simulink model "gm_DUALportRAMinterface_vnl"  (R2024a)
settings: Solver=FixedStepDiscrete  StartTime=0.0  StopTime=2  RelTol=1e-3
undefined symbols (not defined in the file or in its folder): Ts
libraries: hdlsllib x18, simulink x5
settings Model: Creator=Simon  LastModifiedBy=Simon
settings OptimizationCC: BlockReduction=off  ConditionallyExecuteInputs=off  DefaultParameterBehavior=Inlined  InheritOutputTypeSmallerThanSingle=on
settings DebuggingCC: AlgebraicLoopMsg=error  InheritedTsInSrcMsg=none  SingleTaskRateTransMsg=error  UnconnectedInputMsg=warning  UnconnectedOutputMsg=warning  UnconnectedLineMsg=warning
settings HardwareCC: ProdBitPerPointer=32  ProdBitPerSizeT=32  ProdBitPerPtrDiffT=32  ProdLargestAtomicFloat=None  ProdIntDivRoundTo=Undefined  ProdEndianess=Unspecified  ProdWordSize=32  ProdHWDeviceType=ASIC/FPGA->ASIC/FPGA  TargetBitPerPointer=64  TargetBitPerSizeT=64  TargetBitPerPtrDiffT=64  TargetLongLongMode=on  TargetIntDivRoundTo=Zero  TargetEndianess=LittleEndian  TargetWordSize=64  TargetHWDeviceType=Custom Processor->MATLAB Host Computer  ProdEqTarget=off

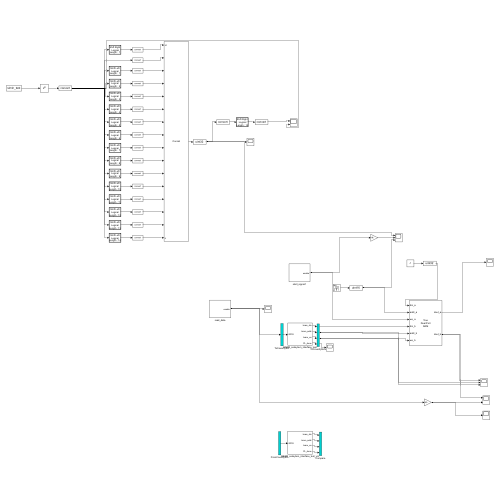
[thumbnail: Simulink's stored preview of the top-level diagram]
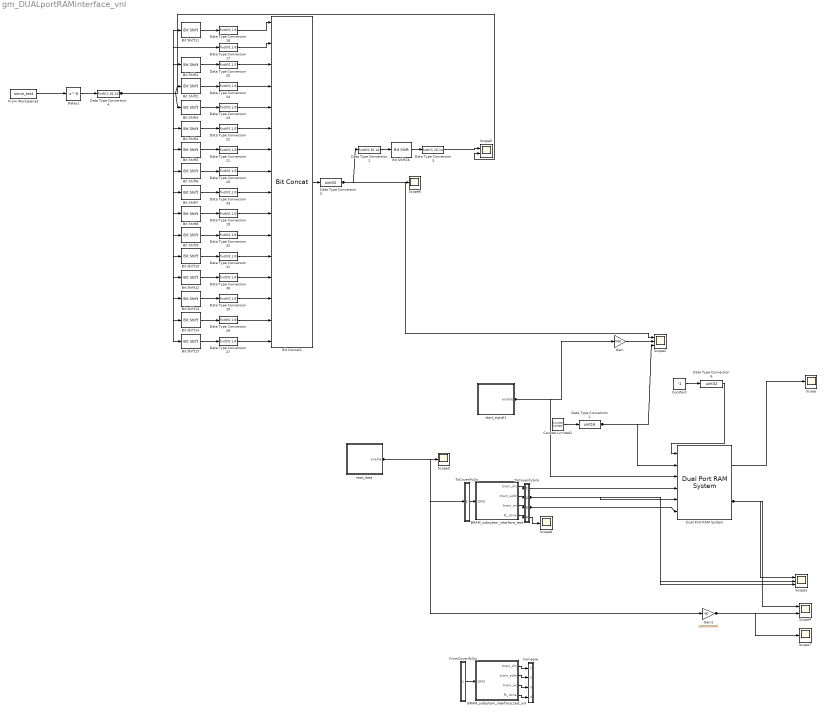
== system gm_DUALportRAMinterface_vnl ==
  BRAM_subsytem_interface_test : Subsystem
  BRAM_subsytem_interface_test_vnl : Subsystem
  Bit Concat1 : hdlsllib/Logic and Bit Operations/Bit Concat  numInputs=16
  Bit Shift1 : hdlsllib/Logic and Bit Operations/Bit Shift  mode=Shift Left Logical  N=1
  Bit Shift10 : hdlsllib/Logic and Bit Operations/Bit Shift  mode=Shift Left Logical  N=10
  Bit Shift11 : hdlsllib/Logic and Bit Operations/Bit Shift  mode=Shift Right Logical  N=1
  Bit Shift12 : hdlsllib/Logic and Bit Operations/Bit Shift  mode=Shift Left Logical  N=11
  Bit Shift13 : hdlsllib/Logic and Bit Operations/Bit Shift  mode=Shift Left Logical  N=12
  Bit Shift14 : hdlsllib/Logic and Bit Operations/Bit Shift  mode=Shift Left Logical  N=13
  Bit Shift15 : hdlsllib/Logic and Bit Operations/Bit Shift  mode=Shift Left Logical  N=14
  Bit Shift16 : hdlsllib/Logic and Bit Operations/Bit Shift  mode=Shift Right Logical  N=14
  Bit Shift2 : hdlsllib/Logic and Bit Operations/Bit Shift  mode=Shift Left Logical  N=2
  Bit Shift3 : hdlsllib/Logic and Bit Operations/Bit Shift  mode=Shift Left Logical  N=3
  Bit Shift4 : hdlsllib/Logic and Bit Operations/Bit Shift  mode=Shift Left Logical  N=4
  Bit Shift5 : hdlsllib/Logic and Bit Operations/Bit Shift  mode=Shift Left Logical  N=5
  Bit Shift6 : hdlsllib/Logic and Bit Operations/Bit Shift  mode=Shift Left Logical  N=6
  Bit Shift7 : hdlsllib/Logic and Bit Operations/Bit Shift  mode=Shift Left Logical  N=7
  Bit Shift8 : hdlsllib/Logic and Bit Operations/Bit Shift  mode=Shift Left Logical  N=8
  Bit Shift9 : hdlsllib/Logic and Bit Operations/Bit Shift  mode=Shift Left Logical  N=9
  Compare : Subsystem
      mask Display: disp('')
  Constant : Constant  Value=-1  SampleTime=-1
  Counter Limited1 : simulink/Sources/Counter Limited  uplimit=7000  tsamp=Ts
  Data Type Conversion1 : DataTypeConversion  OutDataTypeStr=uint16  SaturateOnIntegerOverflow=off  RndMeth=Floor
  Data Type Conversion{17..25,27..33} (16 alike) : DataTypeConversion  OutDataTypeStr=fixdt(0,1,0)  SaturateOnIntegerOverflow=off  RndMeth=Floor
  Data Type Conversion2 : DataTypeConversion  OutDataTypeStr=fixdt(0,30,14)  SaturateOnIntegerOverflow=off  RndMeth=Floor
  Data Type Conversion3 : DataTypeConversion  OutDataTypeStr=fixdt(1,16,14)  SaturateOnIntegerOverflow=off  RndMeth=Floor
  Data Type Conversion4 : DataTypeConversion  OutDataTypeStr=fixdt(1,16,14)  SaturateOnIntegerOverflow=off  RndMeth=Floor
  Data Type Conversion5 : DataTypeConversion  OutDataTypeStr=uint32  SaturateOnIntegerOverflow=off  RndMeth=Floor
  Data Type Conversion6 : DataTypeConversion  OutDataTypeStr=uint32  SaturateOnIntegerOverflow=off  RndMeth=Floor
  Delay1 : Delay  DelayLength=0  InitialCondition=0  SampleTime=Ts
  Dual Port RAM System : hdlsllib/HDL RAMs/Dual Port RAM System  RAMType=True dual port  AsyncRead=off  WriteOutputValue=New data  RAMInitialValue=0  allowBusInputs=off  WritesHaveOutput=on  NumReads=0  NumWrites=1  SimulateUsing=Code generation
  From Workspace3 : FromWorkspace  VariableName=simin_test  SampleTime=Ts
  FromCoverifySrc : Subsystem
      mask Display: disp('')
  Gain : Gain  Gain=7000
  Gain1 : Gain  Gain=1000000000
  Scope{,3,6..8} (5 alike) : Scope
  Scope1 : Scope  NumInputPorts=3
  Scope2 : Scope  NumInputPorts=3
  Scope4 : Scope  NumInputPorts=2
  Scope5 : Scope  NumInputPorts=2
  ToCoverifySink : Subsystem
      mask Display: disp('')
  ToCoverifySrc : Subsystem
      mask Display: disp('')
  read_data : Subsystem
  start_signal1 : Subsystem
  wires:
  Dual Port RAM System/1 -> Scope/1
  Dual Port RAM System/2 -> Scope4/1, Scope1/1
  Counter Limited1/1 -> Data Type Conversion1/1
  Data Type Conversion1/1 -> Scope2/3, Dual Port RAM System/2
  start_signal1/1(enable) -> Dual Port RAM System/3, Gain/1
  Gain/1 -> Scope2/2
  Data Type Conversion3/1 -> Scope5/1
  Bit Shift16/1 -> Data Type Conversion3/1
  Bit Shift1/1 -> Data Type Conversion25/1
  Bit Shift2/1 -> Data Type Conversion24/1
  Data Type Conversion19/1 -> Bit Concat1/10
  Data Type Conversion20/1 -> Bit Concat1/8
  Data Type Conversion30/1 -> Bit Concat1/13
  Data Type Conversion31/1 -> Bit Concat1/12
  Data Type Conversion2/1 -> Bit Shift16/1
  Bit Shift10/1 -> Data Type Conversion31/1
  Bit Shift8/1 -> Data Type Conversion19/1
  Bit Shift12/1 -> Data Type Conversion30/1
  Bit Shift13/1 -> Data Type Conversion29/1
  Bit Concat1/1 -> Data Type Conversion5/1
  Data Type Conversion22/1 -> Bit Concat1/6
  From Workspace3/1 -> Delay1/1
  Bit Shift3/1 -> Data Type Conversion23/1
  Bit Shift7/1 -> Data Type Conversion33/1
  Data Type Conversion5/1 -> Scope2/1, Scope6/1, Data Type Conversion2/1
  Bit Shift14/1 -> Data Type Conversion28/1
  Bit Shift6/1 -> Data Type Conversion20/1
  Bit Shift9/1 -> Data Type Conversion32/1
  Data Type Conversion33/1 -> Bit Concat1/9
  Data Type Conversion21/1 -> Bit Concat1/7
  Data Type Conversion17/1 -> Bit Concat1/2
  Bit Shift15/1 -> Data Type Conversion27/1
  Data Type Conversion28/1 -> Bit Concat1/15
  Data Type Conversion4/1 -> Scope5/2, Bit Shift3/1, Bit Shift4/1, Bit Shift5/1, Bit Shift6/1, Bit Shift7/1, Bit Shift8/1, Bit Shift9/1, Bit Shift10/1, Bit Shift12/1, Bit Shift13/1, Bit Shift15/1, Bit Shift14/1, Bit Shift2/1, Bit Shift1/1, Data Type Conversion17/1, Bit Shift11/1
  Data Type Conversion24/1 -> Bit Concat1/4
  Data Type Conversion32/1 -> Bit Concat1/11
  Delay1/1 -> Data Type Conversion4/1
  Data Type Conversion25/1 -> Bit Concat1/3
  Bit Shift11/1 -> Data Type Conversion18/1
  Data Type Conversion29/1 -> Bit Concat1/14
  Data Type Conversion18/1 -> Bit Concat1/1
  Bit Shift4/1 -> Data Type Conversion22/1
  Data Type Conversion23/1 -> Bit Concat1/5
  Data Type Conversion27/1 -> Bit Concat1/16
  Bit Shift5/1 -> Data Type Conversion21/1
  read_data/1(enable) -> Scope3/1, Gain1/1, ToCoverifySrc/1(in1)
  Constant/1 -> Data Type Conversion6/1
  Data Type Conversion6/1 -> Dual Port RAM System/1
  Gain1/1 -> Scope7/1, Scope4/2
  ToCoverifySrc/1(out1) -> BRAM_subsytem_interface_test/1(GPIO)
  BRAM_subsytem_interface_test/1(bram_din) -> ToCoverifySink/1(in1)
  BRAM_subsytem_interface_test/2(bram_addr) -> ToCoverifySink/2(in2)
  BRAM_subsytem_interface_test/3(bram_en) -> ToCoverifySink/3(in3)
  BRAM_subsytem_interface_test/4(PL_done) -> ToCoverifySink/4(in4)
  ToCoverifySink/1(out1) -> Dual Port RAM System/4
  ToCoverifySink/2(out2) -> Dual Port RAM System/5, Scope1/2
  ToCoverifySink/3(out3) -> Dual Port RAM System/6, Scope1/3
  ToCoverifySink/4(out4) -> Scope8/1
  FromCoverifySrc/1(out1) -> BRAM_subsytem_interface_test_vnl/1(GPIO)
  BRAM_subsytem_interface_test_vnl/1(bram_din) -> Compare/1(in1)
  BRAM_subsytem_interface_test_vnl/2(bram_addr) -> Compare/2(in2)
  BRAM_subsytem_interface_test_vnl/3(bram_en) -> Compare/3(in3)
  BRAM_subsytem_interface_test_vnl/4(PL_done) -> Compare/4(in4)

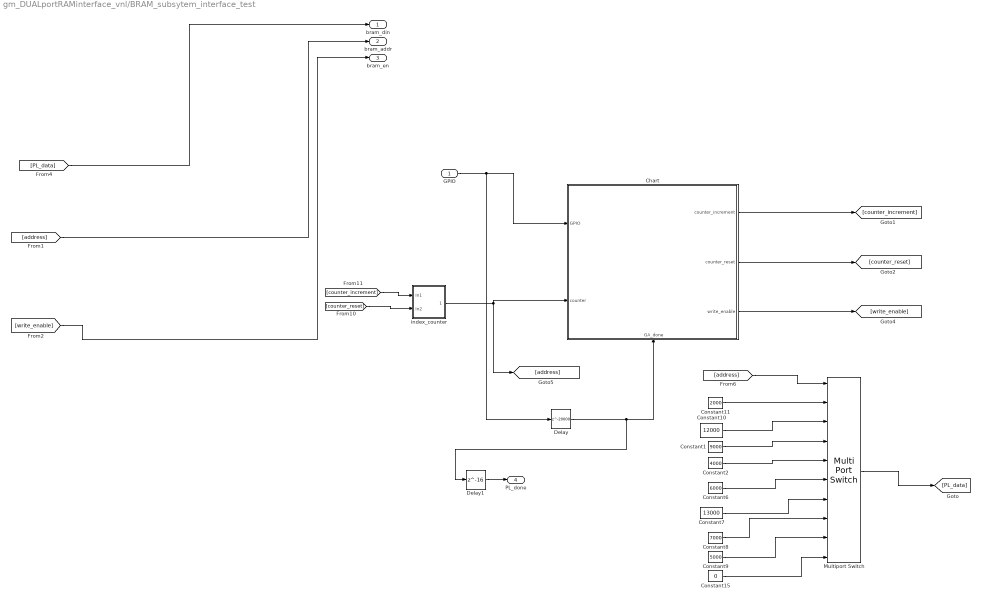
== system gm_DUALportRAMinterface_vnl/BRAM_subsytem_interface_test ==
  GPIO : Inport
  Chart : Stateflow chart  TreatAsAtomicUnit=on
      settings: PortSchema="{\"entries\":[{\"content\":{\"sides\":[{\"content\":{\"connectorIds\":[\"In2\",\"In3\"]},\"type\":\"ConnectorPlacement.EquallySpacedRectSide\",\"uuid\":\"f3ce331f-c708-4668-a9cb-fb327ea74ab5\"},{\"content\":{\"connectorIds\":[\"Out1\",\"Out2\",\"Out3\"],\"side\":\"RIGHT\"},\"type\":\"ConnectorPlacement.EquallySpacedRectSide\",\"uuid\":\"3766927a-abff-497d-9544-2098881ba174\"},{\"content\":{\"side\":\"TOP\"},\"type\":\"ConnectorPlacement.EquallySpacedRectSide\",\"uuid\":\"ebfe3d64-ee7d-4953-a6ba-e7e40988decf\"},{\"content\":{\"connectorIds\":[\"In1\"],\"side\":\"BOTTOM\"},\"type\":\"ConnectorPlacement.EquallySpacedRectSide\",\"uuid\":\"f39ceaf8-4df7-4e40-9de5-da7597831fb4\"}]},\"type\":\"ConnectorPlacement.EquallySpacedConnector\",\"uuid\":\"89f60450-5933-42bb-b72b-5f8ec55483e0\"}],\"packageUris\":[\"http://schema.mathworks.com/mf0/Connector/R2020b\"],\"version\":\"1.0\"}"
  Constant1 : Constant  Value=9000  OutDataTypeStr=uint32  SampleTime=Ts
  Constant10 : Constant  Value=12000  OutDataTypeStr=uint32  SampleTime=Ts
  Constant11 : Constant  Value=2000  OutDataTypeStr=uint32  SampleTime=Ts
  Constant15 : Constant  Value=0  OutDataTypeStr=uint32  SampleTime=Ts
  Constant2 : Constant  Value=4000  OutDataTypeStr=uint32  SampleTime=Ts
  Constant6 : Constant  Value=6000  OutDataTypeStr=uint32  SampleTime=Ts
  Constant7 : Constant  Value=13000  OutDataTypeStr=uint32  SampleTime=Ts
  Constant8 : Constant  Value=7000  OutDataTypeStr=uint32  SampleTime=Ts
  Constant9 : Constant  Value=5000  OutDataTypeStr=uint32  SampleTime=Ts
  Delay : Delay  DelayLength=20000  InitialCondition=0
  Delay1 : Delay  DelayLength=16  InitialCondition=0  SampleTime=Ts
  Multiport Switch : MultiPortSwitch  DataPortOrder=Specify indices  Inputs=8  DataPortIndices={0,1,2,3,4,5,6,7}  DataPortForDefault=Additional data port  DiagnosticForDefault=None  SaturateOnIntegerOverflow=off  InputSameDT=off
  index_counter : Subsystem
  bram_din : Outport
  bram_addr : Outport  Port=2
  bram_en : Outport  Port=3
  PL_done : Outport  Port=4
  wires:
  Multiport Switch/1 -> [PL_data]
  [counter_reset] -> index_counter/2(In2)
  index_counter/1(index_counter) -> Chart/3(counter), [address]
  Constant1/1 -> Multiport Switch/4
  Constant2/1 -> Multiport Switch/5
  [address] -> bram_addr/1
  [counter_increment] -> index_counter/1(In1)
  Constant15/1 -> Multiport Switch/10
  Constant11/1 -> Multiport Switch/2
  [address] -> Multiport Switch/1
  Chart/3(write_enable) -> [write_enable]
  Constant7/1 -> Multiport Switch/7
  GPIO/1 -> Delay/1, Chart/2(GPIO)
  Constant10/1 -> Multiport Switch/3
  Chart/2(counter_reset) -> [counter_reset]
  Chart/1(counter_increment) -> [counter_increment]
  Constant9/1 -> Multiport Switch/9
  Constant8/1 -> Multiport Switch/8
  [PL_data] -> bram_din/1
  Constant6/1 -> Multiport Switch/6
  [write_enable] -> bram_en/1
  Delay/1 -> Delay1/1, Chart/1(GA_done)
  Delay1/1 -> PL_done/1

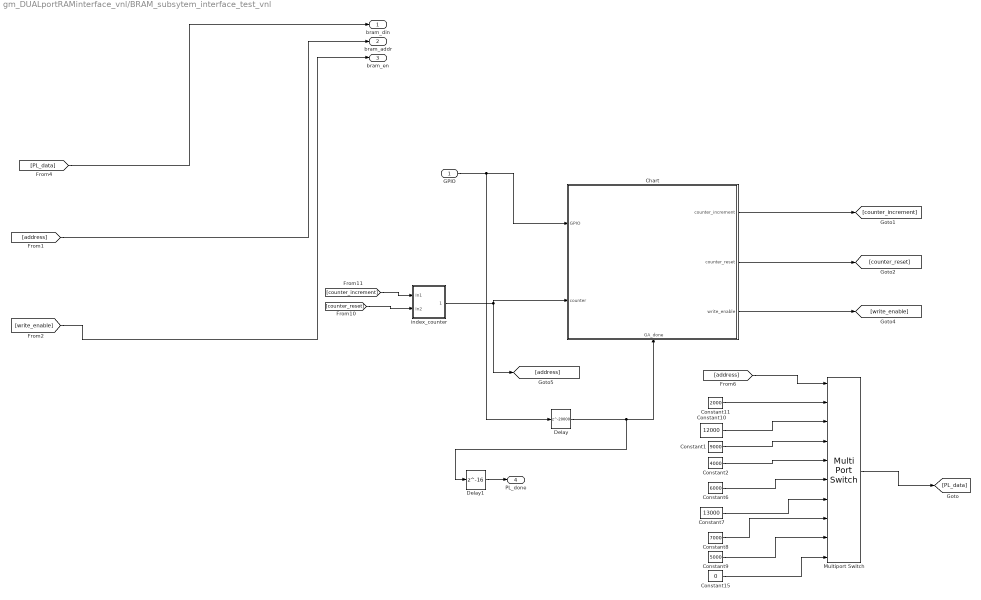
== system gm_DUALportRAMinterface_vnl/BRAM_subsytem_interface_test_vnl ==
  GPIO : Inport
  Chart : Stateflow chart  TreatAsAtomicUnit=on
      settings: PortSchema="{\"entries\":[{\"content\":{\"sides\":[{\"content\":{\"connectorIds\":[\"In2\",\"In3\"]},\"type\":\"ConnectorPlacement.EquallySpacedRectSide\",\"uuid\":\"f3ce331f-c708-4668-a9cb-fb327ea74ab5\"},{\"content\":{\"connectorIds\":[\"Out1\",\"Out2\",\"Out3\"],\"side\":\"RIGHT\"},\"type\":\"ConnectorPlacement.EquallySpacedRectSide\",\"uuid\":\"3766927a-abff-497d-9544-2098881ba174\"},{\"content\":{\"side\":\"TOP\"},\"type\":\"ConnectorPlacement.EquallySpacedRectSide\",\"uuid\":\"ebfe3d64-ee7d-4953-a6ba-e7e40988decf\"},{\"content\":{\"connectorIds\":[\"In1\"],\"side\":\"BOTTOM\"},\"type\":\"ConnectorPlacement.EquallySpacedRectSide\",\"uuid\":\"f39ceaf8-4df7-4e40-9de5-da7597831fb4\"}]},\"type\":\"ConnectorPlacement.EquallySpacedConnector\",\"uuid\":\"89f60450-5933-42bb-b72b-5f8ec55483e0\"}],\"packageUris\":[\"http://schema.mathworks.com/mf0/Connector/R2020b\"],\"version\":\"1.0\"}"
  Constant1 : Constant  Value=9000  OutDataTypeStr=uint32  SampleTime=Ts
  Constant10 : Constant  Value=12000  OutDataTypeStr=uint32  SampleTime=Ts
  Constant11 : Constant  Value=2000  OutDataTypeStr=uint32  SampleTime=Ts
  Constant15 : Constant  Value=0  OutDataTypeStr=uint32  SampleTime=Ts
  Constant2 : Constant  Value=4000  OutDataTypeStr=uint32  SampleTime=Ts
  Constant6 : Constant  Value=6000  OutDataTypeStr=uint32  SampleTime=Ts
  Constant7 : Constant  Value=13000  OutDataTypeStr=uint32  SampleTime=Ts
  Constant8 : Constant  Value=7000  OutDataTypeStr=uint32  SampleTime=Ts
  Constant9 : Constant  Value=5000  OutDataTypeStr=uint32  SampleTime=Ts
  Delay : Delay  DelayLength=20000  InitialCondition=0
  Delay1 : Delay  DelayLength=16  InitialCondition=0  SampleTime=Ts
  Multiport Switch : MultiPortSwitch  DataPortOrder=Specify indices  Inputs=8  DataPortIndices={0,1,2,3,4,5,6,7}  DataPortForDefault=Additional data port  DiagnosticForDefault=None  SaturateOnIntegerOverflow=off  InputSameDT=off
  index_counter : Subsystem
  bram_din : Outport
  bram_addr : Outport  Port=2
  bram_en : Outport  Port=3
  PL_done : Outport  Port=4
  wires:
  Delay1/1 -> PL_done/1
  Delay/1 -> Chart/1(GA_done), Delay1/1
  [write_enable] -> bram_en/1
  Constant6/1 -> Multiport Switch/6
  [PL_data] -> bram_din/1
  Constant8/1 -> Multiport Switch/8
  Constant9/1 -> Multiport Switch/9
  Chart/1(counter_increment) -> [counter_increment]
  Chart/2(counter_reset) -> [counter_reset]
  Constant10/1 -> Multiport Switch/3
  GPIO/1 -> Chart/2(GPIO), Delay/1
  Constant7/1 -> Multiport Switch/7
  Chart/3(write_enable) -> [write_enable]
  [address] -> Multiport Switch/1
  Constant11/1 -> Multiport Switch/2
  Constant15/1 -> Multiport Switch/10
  [counter_increment] -> index_counter/1(In1)
  [address] -> bram_addr/1
  Constant2/1 -> Multiport Switch/5
  Constant1/1 -> Multiport Switch/4
  index_counter/1(index_counter) -> [address], Chart/3(counter)
  [counter_reset] -> index_counter/2(In2)
  Multiport Switch/1 -> [PL_data]

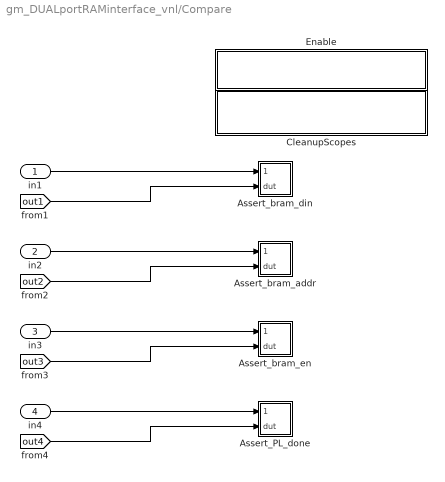
== system gm_DUALportRAMinterface_vnl/Compare ==
  in1 : Inport
  in2 : Inport  Port=2
  in3 : Inport  Port=3
  in4 : Inport  Port=4
  Assert_PL_done : Subsystem
      settings: LibrarySourceBlock=hdlmdlgenlib/AssertEq
  Assert_bram_addr : Subsystem
      settings: LibrarySourceBlock=hdlmdlgenlib/AssertEq
  Assert_bram_din : Subsystem
      settings: LibrarySourceBlock=hdlmdlgenlib/AssertEq
  Assert_bram_en : Subsystem
      settings: LibrarySourceBlock=hdlmdlgenlib/AssertEq
  CleanupScopes : Subsystem
      settings: OpenFcn=|
      | blkName = gcb; %self block
      | idx = regexp(blkName, '/CleanupScopes$', 'once');
      | blkParent = blkName(1:idx-1);
      | blks=find_system(blkParent, 'LookUnderMasks', 'all','blocktype', 'Scope');
      | for itr = 1:length(blks)
      | 	 hScopeCfg = get_param(blks{itr},'ScopeConfiguration');
      | 	 hScopeCfg.Visible = ~ hScopeCfg.Visible;
      | end
      | drawnow;
      mask Display: fprintf(message('hdlcoder:cosim:vnl_dblclick').getString());
  Enable : Subsystem
      settings: OpenFcn=|
      | blkName = gcb;
      | idx = regexp(blkName, '/Enable$', 'once');
      | blkParent = blkName(1:idx-1);
      | blks=find_system(blkParent, 'LookUnderMasks', 'all','blocktype', 'Assertion');
      | e = get_param(blks{1}, 'Enabled');
      | if strcmp(e, 'on'), f= 'off';, else, f = 'on';, end
      | for ii=1:length(blks), set_param(blks{ii}, 'Enabled', f);, end
      | set_param(gcb, 'MaskDisplay',['fprintf(message(''hdlcoder:cosim:vnl_dblclick_assertions'',','''',upper(e),'''',').getString())']);
      mask Display: fprintf(message('hdlcoder:cosim:vnl_dblclick_assertions','OFF').getString());
  wires:
  in1/1 -> Assert_bram_din/1(cosim)
  [out1] -> Assert_bram_din/2(dut)
  in2/1 -> Assert_bram_addr/1(cosim)
  [out2] -> Assert_bram_addr/2(dut)
  in3/1 -> Assert_bram_en/1(cosim)
  [out3] -> Assert_bram_en/2(dut)
  in4/1 -> Assert_PL_done/1(cosim)
  [out4] -> Assert_PL_done/2(dut)

== system gm_DUALportRAMinterface_vnl/FromCoverifySrc ==
  out1 : Outport
  wires:
  [in1] -> out1/1

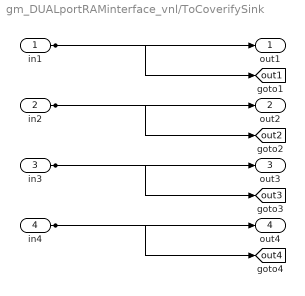
== system gm_DUALportRAMinterface_vnl/ToCoverifySink ==
  in1 : Inport
  in2 : Inport  Port=2
  in3 : Inport  Port=3
  in4 : Inport  Port=4
  out1 : Outport
  out2 : Outport  Port=2
  out3 : Outport  Port=3
  out4 : Outport  Port=4
  tag scope: out1=global, out2=global, out3=global, out4=global
  wires:
  in1/1 -> out1/1, [out1]
  in2/1 -> out2/1, [out2]
  in3/1 -> out3/1, [out3]
  in4/1 -> out4/1, [out4]

== system gm_DUALportRAMinterface_vnl/ToCoverifySrc ==
  in1 : Inport
  out1 : Outport
  tag scope: in1=global
  wires:
  in1/1 -> out1/1, [in1]

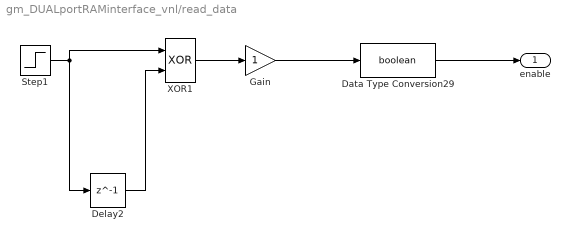
== system gm_DUALportRAMinterface_vnl/read_data ==
  Data Type Conversion29 : DataTypeConversion  OutDataTypeStr=boolean  SaturateOnIntegerOverflow=off  RndMeth=Floor
  Delay2 : Delay  DelayLength=1  InitialCondition=0  SampleTime=Ts
  Gain : Gain
  Step1 : Step  Time=Ts*7000  SampleTime=Ts
  XOR1 : Logic  Operator=XOR  IconShape=distinctive  AllPortsSameDT=off  OutDataTypeStr=boolean
  enable : Outport
  wires:
  XOR1/1 -> Gain/1
  Step1/1 -> Delay2/1, XOR1/1
  Delay2/1 -> XOR1/2
  Gain/1 -> Data Type Conversion29/1
  Data Type Conversion29/1 -> enable/1

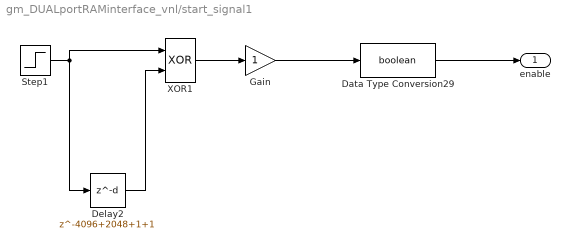
== system gm_DUALportRAMinterface_vnl/start_signal1 ==
  Data Type Conversion29 : DataTypeConversion  OutDataTypeStr=boolean  SaturateOnIntegerOverflow=off  RndMeth=Floor
  Delay2 : Delay  DelayLength=4096+2048+1+1  InitialCondition=0  SampleTime=Ts
  Gain : Gain
  Step1 : Step  Time=Ts*0  SampleTime=Ts
  XOR1 : Logic  Operator=XOR  IconShape=distinctive  AllPortsSameDT=off  OutDataTypeStr=boolean
  enable : Outport
  wires:
  Data Type Conversion29/1 -> enable/1
  Gain/1 -> Data Type Conversion29/1
  Delay2/1 -> XOR1/2
  Step1/1 -> XOR1/1, Delay2/1
  XOR1/1 -> Gain/1

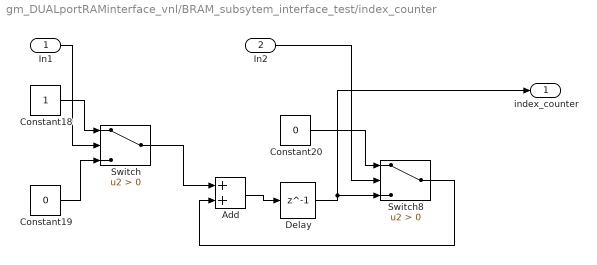
== system gm_DUALportRAMinterface_vnl/BRAM_subsytem_interface_test/index_counter ==
  In1 : Inport
  In2 : Inport  Port=2
  Add : Sum  OutDataTypeStr=Inherit: Same as first input
  Constant18 : Constant  OutDataTypeStr=fixdt(0,16,0)  SampleTime=Ts
  Constant19 : Constant  Value=0  OutDataTypeStr=fixdt(0,16,0)  SampleTime=Ts
  Constant20 : Constant  Value=0  OutDataTypeStr=uint16  SampleTime=Ts
  Delay : Delay  DelayLength=1  InitialCondition=0  SampleTime=Ts
  Switch : Switch  Criteria=u2 > Threshold  SaturateOnIntegerOverflow=off  InputSameDT=off  OutDataTypeStr=Inherit: Same as first input
  Switch8 : Switch  Criteria=u2 > Threshold  SaturateOnIntegerOverflow=off  InputSameDT=off  OutDataTypeStr=Inherit: Same as first input
  index_counter : Outport
  wires:
  Constant19/1 -> Switch/3
  Switch8/1 -> Add/2
  Switch/1 -> Add/1
  Delay/1 -> index_counter/1, Switch8/3
  In2/1 -> Switch8/2
  Add/1 -> Delay/1
  Constant20/1 -> Switch8/1
  Constant18/1 -> Switch/1
  In1/1 -> Switch/2

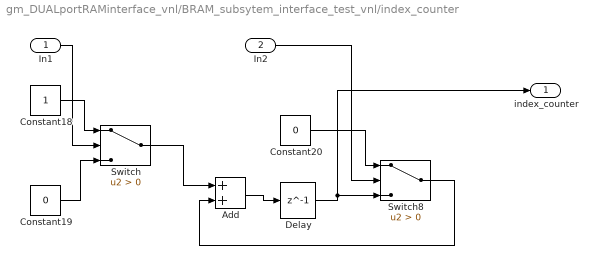
== system gm_DUALportRAMinterface_vnl/BRAM_subsytem_interface_test_vnl/index_counter ==
  In1 : Inport
  In2 : Inport  Port=2
  Add : Sum  OutDataTypeStr=Inherit: Same as first input
  Constant18 : Constant  OutDataTypeStr=fixdt(0,16,0)  SampleTime=Ts
  Constant19 : Constant  Value=0  OutDataTypeStr=fixdt(0,16,0)  SampleTime=Ts
  Constant20 : Constant  Value=0  OutDataTypeStr=uint16  SampleTime=Ts
  Delay : Delay  DelayLength=1  InitialCondition=0  SampleTime=Ts
  Switch : Switch  Criteria=u2 > Threshold  SaturateOnIntegerOverflow=off  InputSameDT=off  OutDataTypeStr=Inherit: Same as first input
  Switch8 : Switch  Criteria=u2 > Threshold  SaturateOnIntegerOverflow=off  InputSameDT=off  OutDataTypeStr=Inherit: Same as first input
  index_counter : Outport
  wires:
  In1/1 -> Switch/2
  Constant18/1 -> Switch/1
  Constant20/1 -> Switch8/1
  Add/1 -> Delay/1
  In2/1 -> Switch8/2
  Delay/1 -> Switch8/3, index_counter/1
  Switch/1 -> Add/1
  Switch8/1 -> Add/2
  Constant19/1 -> Switch/3

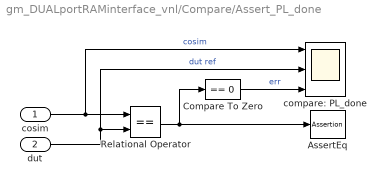
== system gm_DUALportRAMinterface_vnl/Compare/Assert_PL_done ==
  cosim : Inport
  dut : Inport  Port=2
  AssertEq : Assertion  StopWhenAssertionFail=off
  Compare To Zero : simulink/Logic and Bit Operations/Compare To Zero  relop===  OutDataTypeStr=boolean
  Relational Operator : RelationalOperator  Operator===  OutDataTypeStr=boolean  InputSameDT=off
  compare: PL_done : Scope  NumInputPorts=3
  wires:
  Compare To Zero/1 -> compare: PL_done/3  "err"
  Relational Operator/1 -> Compare To Zero/1, AssertEq/1
  cosim/1 -> compare: PL_done/1, Relational Operator/1  "cosim"
  dut/1 -> compare: PL_done/2, Relational Operator/2  "dut ref"

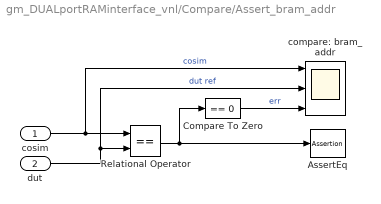
== system gm_DUALportRAMinterface_vnl/Compare/Assert_bram_addr ==
  cosim : Inport
  dut : Inport  Port=2
  AssertEq : Assertion  StopWhenAssertionFail=off
  Compare To Zero : simulink/Logic and Bit Operations/Compare To Zero  relop===  OutDataTypeStr=boolean
  Relational Operator : RelationalOperator  Operator===  OutDataTypeStr=boolean  InputSameDT=off
  compare: bram_addr : Scope  NumInputPorts=3
  wires:
  Compare To Zero/1 -> compare: bram_addr/3  "err"
  Relational Operator/1 -> Compare To Zero/1, AssertEq/1
  cosim/1 -> compare: bram_addr/1, Relational Operator/1  "cosim"
  dut/1 -> compare: bram_addr/2, Relational Operator/2  "dut ref"

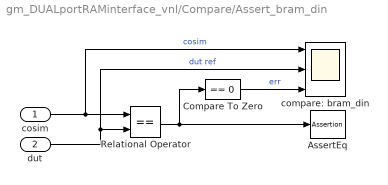
== system gm_DUALportRAMinterface_vnl/Compare/Assert_bram_din ==
  cosim : Inport
  dut : Inport  Port=2
  AssertEq : Assertion  StopWhenAssertionFail=off
  Compare To Zero : simulink/Logic and Bit Operations/Compare To Zero  relop===  OutDataTypeStr=boolean
  Relational Operator : RelationalOperator  Operator===  OutDataTypeStr=boolean  InputSameDT=off
  compare: bram_din : Scope  NumInputPorts=3
  wires:
  Compare To Zero/1 -> compare: bram_din/3  "err"
  Relational Operator/1 -> Compare To Zero/1, AssertEq/1
  cosim/1 -> compare: bram_din/1, Relational Operator/1  "cosim"
  dut/1 -> compare: bram_din/2, Relational Operator/2  "dut ref"

== system gm_DUALportRAMinterface_vnl/Compare/Assert_bram_en ==
  cosim : Inport
  dut : Inport  Port=2
  AssertEq : Assertion  StopWhenAssertionFail=off
  Compare To Zero : simulink/Logic and Bit Operations/Compare To Zero  relop===  OutDataTypeStr=boolean
  Relational Operator : RelationalOperator  Operator===  OutDataTypeStr=boolean  InputSameDT=off
  compare: bram_en : Scope  NumInputPorts=3
  wires:
  Compare To Zero/1 -> compare: bram_en/3  "err"
  Relational Operator/1 -> Compare To Zero/1, AssertEq/1
  cosim/1 -> compare: bram_en/1, Relational Operator/1  "cosim"
  dut/1 -> compare: bram_en/2, Relational Operator/2  "dut ref"

== system gm_DUALportRAMinterface_vnl/Compare/CleanupScopes ==

== system gm_DUALportRAMinterface_vnl/Compare/Enable ==

== stateflow chart gm_DUALportRAMinterface_vnl/BRAM_subsytem_interface_test_vnl/Chart ==
  settings: executeAtInitialization=1
  state initial_wait_state
    entry:
    counter_increment = false;
    counter_reset = true;
    write_enable = false;
  state PL_read_data
    entry:
    counter_increment = true;
    counter_reset = false;
    write_enable = false;
  state wait_for_GA_done
    entry:
    counter_increment = false;
    counter_reset = true;
    write_enable = false;
  state reset_state
    entry:
    counter_increment = false;
    counter_reset = true;
    write_enable = false;
  state PL_write_data_back
    entry:
    counter_increment = true;
    counter_reset = false;
    write_enable = true;
  (default) -> initial_wait_state
  initial_wait_state -> PL_read_data : [GPIO == 1]
  reset_state -> initial_wait_state
  PL_read_data -> wait_for_GA_done : [counter == 4096+2048+1]
  wait_for_GA_done -> PL_write_data_back : [GA_done == 1]
  PL_write_data_back -> reset_state : [counter == 8]
  data: GA_done input boolean; GPIO input; counter input; counter_increment output boolean; counter_reset output boolean; write_enable output boolean

== stateflow chart gm_DUALportRAMinterface_vnl/BRAM_subsytem_interface_test/Chart ==
  settings: executeAtInitialization=1
  state initial_wait_state
    entry:
    counter_increment = false;
    counter_reset = true;
    write_enable = false;
  state PL_read_data
    entry:
    counter_increment = true;
    counter_reset = false;
    write_enable = false;
  state wait_for_GA_done
    entry:
    counter_increment = false;
    counter_reset = true;
    write_enable = false;
  state reset_state
    entry:
    counter_increment = false;
    counter_reset = true;
    write_enable = false;
  state PL_write_data_back
    entry:
    counter_increment = true;
    counter_reset = false;
    write_enable = true;
  (default) -> initial_wait_state
  initial_wait_state -> PL_read_data : [GPIO == 1]
  reset_state -> initial_wait_state
  PL_read_data -> wait_for_GA_done : [counter == 4096+2048+1]
  wait_for_GA_done -> PL_write_data_back : [GA_done == 1]
  PL_write_data_back -> reset_state : [counter == 8]
  data: GA_done input boolean; GPIO input; counter input; counter_increment output boolean; counter_reset output boolean; write_enable output boolean
